simulink model "lege_de_atingere"  (R2018b)
settings: Solver=VariableStepAuto  StartTime=0.0  StopTime=10  RelTol=1e-3
values from neighbouring files (symbols this model uses):
  J = 0.71e-3    (= 0.00071)    [Date.m]
  ke = 0.33    [Date.m]
  km = 0.33    [Date.m]
  kp = 35    [Date.m]
  La = 14.28e-3    (= 0.01428)    [Date.m]
  Ra = 4.2    [Date.m]
settings Model: Creator=adrianb3  LastModifiedBy=adrianb3

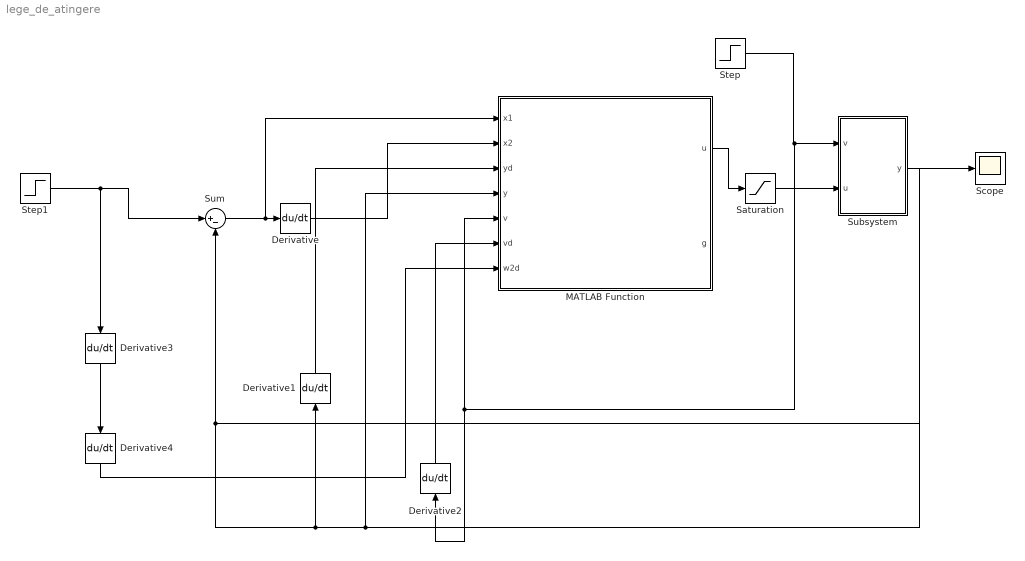
== system lege_de_atingere ==
  Derivative{,1..4} (5 alike) : Derivative
  MATLAB Function : MATLAB Function  TreatAsAtomicUnit=on
  Saturation : Saturate  UpperLimit=30  LowerLimit=-30
  Scope : Scope
  Step : Step  Time=0.6  After=-12  SampleTime=0
  Step1 : Step  Time=0  After=20  SampleTime=0
  Subsystem : Subsystem
  Sum : Sum  Inputs=|+-
  wires:
  Step/1 -> Derivative2/1, MATLAB Function/5(v), Subsystem/1(v)
  MATLAB Function/1(u) -> Saturation/1
  Step1/1 -> Sum/1, Derivative3/1
  Subsystem/1(y) -> MATLAB Function/4(y), Derivative1/1, Sum/2, Scope/1
  Sum/1 -> MATLAB Function/1(x1), Derivative/1
  Derivative/1 -> MATLAB Function/2(x2)
  Derivative1/1 -> MATLAB Function/3(yd)
  Derivative2/1 -> MATLAB Function/6(vd)
  Derivative3/1 -> Derivative4/1
  Derivative4/1 -> MATLAB Function/7(w2d)
  Saturation/1 -> Subsystem/2(u)

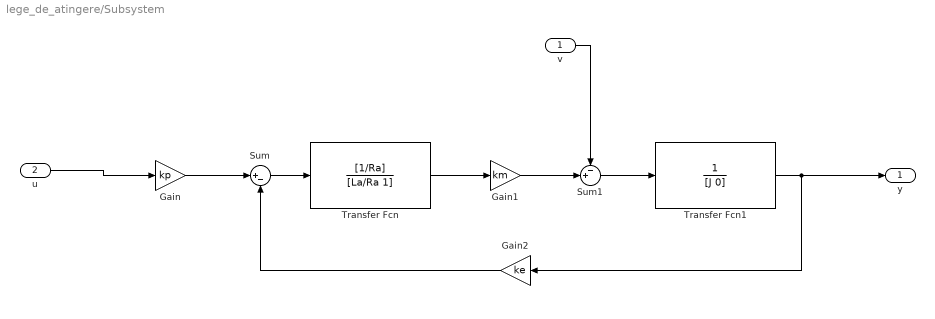
== system lege_de_atingere/Subsystem ==
  v : Inport
  u : Inport  Port=2
  Gain : Gain  Gain=kp
  Gain1 : Gain  Gain=km
  Gain2 : Gain  Gain=ke
  Sum : Sum  Inputs=|+-
  Sum1 : Sum  Inputs=-+|
  Transfer Fcn : TransferFcn  Numerator=[1/Ra]  Denominator=[La/Ra 1]
  Transfer Fcn1 : TransferFcn  Denominator=[J 0]
  y : Outport
  wires:
  Sum/1 -> Transfer Fcn/1
  Sum1/1 -> Transfer Fcn1/1
  Transfer Fcn/1 -> Gain1/1
  Gain1/1 -> Sum1/2
  v/1 -> Sum1/1
  Transfer Fcn1/1 -> y/1, Gain2/1
  u/1 -> Gain/1
  Gain/1 -> Sum/1
  Gain2/1 -> Sum/2

== matlab function lege_de_atingere/MATLAB Function ==
  data: x1 input; u output; x2 input; g output; yd input; y input; v input; vd input; w2d input
function [u, g] = lda(x1, x2, yd, y, v, vd, w2d)
km=0.33;
Ra=4.2;
ke=0.33;
La=14.28e-3;
J=0.71e-3;
kp=35;
c=240;
b=-(kp*km)/(La*J);
z=(-Ra/La)*yd-((km*ke)/(La*J)) * y-(Ra/(La*J))*v - (1/J)*vd;
%z=-294.1176 * yd - 1.0741e+04*y-1.4085e+03*vd-4.142e+05*v;
k = 28000000;
g=c*x1+x2;
u=b^-1 * (w2d - c*x2 - z) -( b^(-1) * k * sign(g));
end
